simulink model "Accoppiato_percorso_lineare"  (R2020a)
settings: Solver=VariableStepAuto  StartTime=0.0  StopTime=1000  RelTol=1e-3
values from neighbouring files (symbols this model uses):
  Ag = 1    [completeLinearSimulation.m]
  Al = 1    [completeLinearSimulation.m]
  Cd = 1.2    [completeLinearSimulation.m]
  Cl = 0.3    [completeLinearSimulation.m]
  g = 9.81    [completeLinearSimulation.m]
  h = 1    [completeLinearSimulation.m]
  i_e = 100    [completeLinearSimulation.m]
  id1_ref = 0    [completeLinearSimulation.m]
  id2_ref = 0    [completeLinearSimulation.m]
  ig1_init = 0    [completeLinearSimulation.m]
  ig3_init = 0    [completeLinearSimulation.m]
  ig4_init = 0    [completeLinearSimulation.m]
  iq1_ref = (Fx1_ref)/((3/2)*(pi/tau)*(Ld*(M/Ld)*i_e))    (= 482.136730936)    [completeLinearSimulation.m]
  iq2_ref = (Fx2_ref)/((3/2)*(pi/tau)*(Ld*(M/Ld)*i_e))    (= 482.136730936)    [completeLinearSimulation.m]
  Jx = 296*10^3    (= 296000)    [completeLinearSimulation.m]
  Jy = 2853*10^3    (= 2853000)    [completeLinearSimulation.m]
  Jz = 2853*10^3    (= 2853000)    [completeLinearSimulation.m]
  Ky = lqr(Ay,By,Qy,Rry)    [completeLinearSimulation.m]
  Kz = lqr(Az,Bz,Qz,Rrz)    [completeLinearSimulation.m]
  l = 8    [completeLinearSimulation.m]
  Ld = 0.06    [completeLinearSimulation.m]
  Lq = 0.06    [completeLinearSimulation.m]
  M = 0.1    [completeLinearSimulation.m]
  m = 60000    [completeLinearSimulation.m]
  mu0 = 1.25*10^-6    (= 1.25e-06)    [completeLinearSimulation.m]
  Ng = 500    [completeLinearSimulation.m]
  Nr = 300    [completeLinearSimulation.m]
  p = 3    [completeLinearSimulation.m]
  PHI12 = eval(PHI)    [completeLinearSimulation.m]
  PHI20 = eval(PHI)    [completeLinearSimulation.m]
  PHI4 = eval(PHI)    [completeLinearSimulation.m]
  phi_init = 0    [completeLinearSimulation.m]
  PHIc = eval(int21)    [completeLinearSimulation.m]
  PHIf = eval(int11)    [completeLinearSimulation.m]
  PHIr = eval(int31)    [completeLinearSimulation.m]
  phiy = 0    [completeLinearSimulation.m]
  psi_init = 0    [completeLinearSimulation.m]
  ql_init = 0    [completeLinearSimulation.m]
  qv_init = 0    [completeLinearSimulation.m]
  Ra = 0    [completeLinearSimulation.m]
  radius = 0    [completeLinearSimulation.m]
  Rg = 100    [completeLinearSimulation.m]
  rho = 1.225    [completeLinearSimulation.m]
  Rx = 1.04    [completeLinearSimulation.m]
  Rz = 100    [completeLinearSimulation.m]
  Sa = 13    [completeLinearSimulation.m]
  Ss = 13    [completeLinearSimulation.m]
  tau = 1    [completeLinearSimulation.m]
  theta_init = 0    [completeLinearSimulation.m]
  vql_init = 0    [completeLinearSimulation.m]
  vqv_init = 0    [completeLinearSimulation.m]
  Vref_x = [Vq1_ref; Vd1_ref; Vq2_ref; Vd2_ref]    [completeLinearSimulation.m]
  Vref_y = [ Vg1; Vg2; Vg3; Vg4; Vg5; Vg6]    [completeLinearSimulation.m]
  Vref_z = [Vr1_ref; Vr2_ref; Vr3_ref; Vr4_ref; Vr5_ref; Vr6_ref]    [completeLinearSimulation.m]
  vx = 400/3.6    (= 111.111111111)    [completeLinearSimulation.m]
  vy_init = 0    [completeLinearSimulation.m]
  w = eval(omega_1)    [completeLinearSimulation.m]
  wpsi_init = 0    [completeLinearSimulation.m]
  xA = 12    [completeLinearSimulation.m]
  xB = 8    [completeLinearSimulation.m]
  Xref = [iq1_ref; id1_ref; iq2_ref; id2_ref; xdot_ref]    [completeLinearSimulation.m]
  y_init = 0.01    [completeLinearSimulation.m]
  yB = 2    [completeLinearSimulation.m]
  ymax = 0.02    [completeLinearSimulation.m]
  Yref = [y_ref; vy_ref; psi_ref; wpsi_ref; ig_ref; ig_ref; ig_ref; ig_ref; ig_ref; ig_ref; ql_ref; vql_ref]    [completeLinearSimulation.m]
  zA = 0.5    [completeLinearSimulation.m]
  zB = -0.5    [completeLinearSimulation.m]
  zi_rip = 0.05    [completeLinearSimulation.m]
  Zref = [z_ref zdot_ref phi_ref phidot_ref theta_ref thetadot_ref ir1_ref ir2_ref ir3_ref ir4_ref ir5_ref ir6_ref qv_ref vqv_ref].'    [completeLinearSimulation.m]
undefined symbols (not defined in the file or in its folder): Kx
settings Model: Creator=Federico  LastModifiedBy=Federico

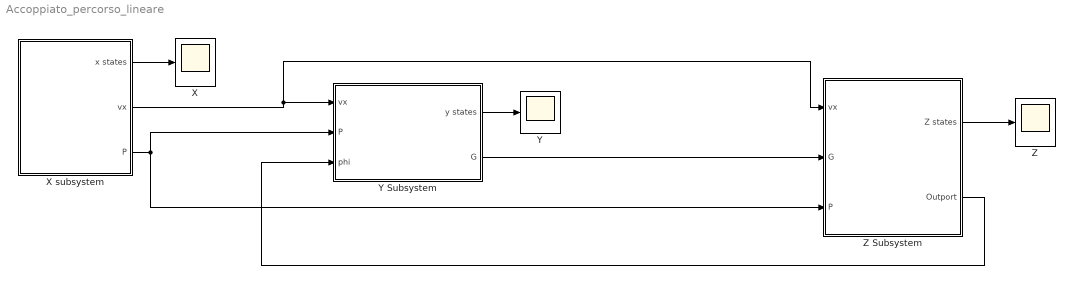
== system Accoppiato_percorso_lineare ==
  X : Scope
  X subsystem : Subsystem
  Y : Scope
  Y Subsystem : Subsystem
  Z : Scope
  Z Subsystem : Subsystem
  wires:
  X subsystem/1(x states) -> X/1
  X subsystem/3(P) -> Z Subsystem/3(P), Y Subsystem/2(P)
  X subsystem/2(vx) -> Z Subsystem/1(vx), Y Subsystem/1(vx)
  Y Subsystem/2(G) -> Z Subsystem/2(G)
  Y Subsystem/1(y states) -> Y/1
  Z Subsystem/1(Z states) -> Z/1
  Z Subsystem/2(Outport) -> Y Subsystem/3(phi)

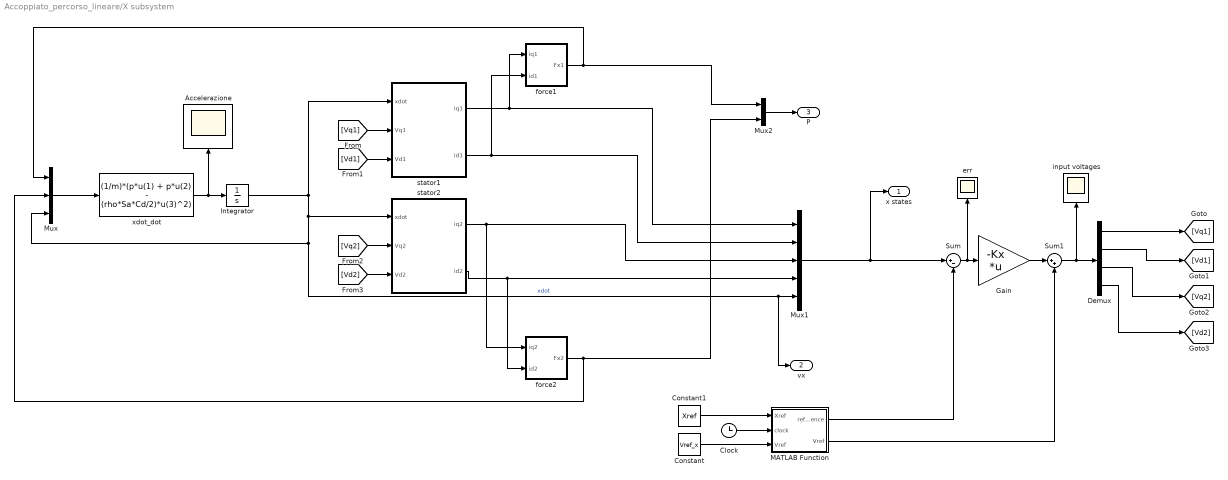
== system Accoppiato_percorso_lineare/X subsystem ==
  Accelerazione : Scope
  Clock : Clock
  Constant : Constant  Value=Vref_x
  Constant1 : Constant  Value=Xref
  Demux : Demux
  Gain : Gain  Gain=-Kx  Multiplication=Matrix(K*u)
  Integrator : Integrator
  MATLAB Function : MATLAB Function  TreatAsAtomicUnit=on
  Mux : Mux  Inputs=3
  Mux1 : Mux  Inputs=5
  Mux2 : Mux  Inputs=2
  Sum : Sum  Inputs=|+-
  Sum1 : Sum  Inputs=|++
  err : Scope
  force1 : Subsystem
  force2 : Subsystem
  input voltages : Scope
  stator1 : Subsystem
  stator2 : Subsystem
  xdot_dot : Fcn  Expr=(1/m)*(p*u(1) + p*u(2) - (rho*Sa*Cd/2)*u(3)^2)
  x states : Outport
  vx : Outport  Port=2
  P : Outport  Port=3
  wires:
  MATLAB Function/1(reference) -> Sum/2
  stator1/2(id1) -> Mux1/2, force1/2(id1)
  Sum1/1 -> Demux/1, input voltages/1
  Integrator/1 -> Mux/3, vx/1, Mux1/5, stator2/1(xdot), stator1/1(xdot)  "xdot"
  stator2/2(id2) -> force2/2(id2), Mux1/4
  [Vd2] -> stator2/3(Vd2)
  xdot_dot/1 -> Integrator/1, Accelerazione/1
  Demux/4 -> [Vd2]
  force1/1(Fx1) -> Mux2/1, Mux/1
  Mux1/1 -> Sum/1, x states/1
  Gain/1 -> Sum1/1
  MATLAB Function/2(Vref) -> Sum1/2
  Mux/1 -> xdot_dot/1
  Constant1/1 -> MATLAB Function/1(Xref)
  Sum/1 -> err/1, Gain/1
  Demux/1 -> [Vq1]
  stator1/1(iq1) -> Mux1/1, force1/1("iq1 ")
  Clock/1 -> MATLAB Function/2(clock)
  stator2/1(iq2) -> force2/1("iq2 "), Mux1/3
  Demux/3 -> [Vq2]
  [Vq2] -> stator2/2(Vq2)
  Constant/1 -> MATLAB Function/3("Vref ")
  Demux/2 -> [Vd1]
  [Vq1] -> stator1/2(Vq1)
  [Vd1] -> stator1/3(Vd1)
  force2/1(Fx2) -> Mux/2, Mux2/2
  Mux2/1 -> P/1

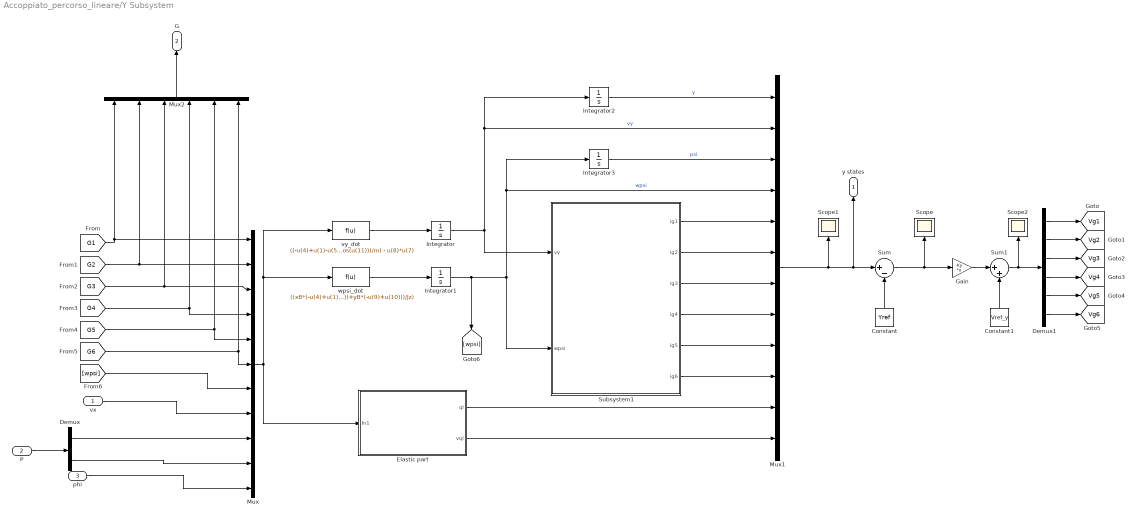
== system Accoppiato_percorso_lineare/Y Subsystem ==
  vx : Inport
  P : Inport  Port=2
  phi : Inport  Port=3
  Constant : Constant  Value=Yref
  Constant1 : Constant  Value=Vref_y
  Demux : Demux  Outputs=2
  Demux1 : Demux  Outputs=6
  Elastic part : Subsystem
  Gain : Gain  Gain=-Ky  Multiplication=Matrix(K*u)
  Integrator : Integrator  InitialCondition=vy_init
  Integrator1 : Integrator  InitialCondition=wpsi_init
  Integrator2 : Integrator  InitialCondition=y_init
  Integrator3 : Integrator  InitialCondition=psi_init
  Mux : Mux  Inputs=11
  Mux1 : Mux  Inputs=12
  Mux2 : Mux  Inputs=6
  Scope : Scope
  Scope1 : Scope
  Scope2 : Scope
  Subsystem1 : Subsystem
  Sum : Sum  Inputs=|+-
  Sum1 : Sum  Inputs=|++
  vy_dot : Fcn  Expr=((-u(4)+u(1)-u(5)+u(2)-u(6)+u(3)+m*g*sin(u(11))-m*Ra*(u(7)^2)*cos(u(11)))/m) - u(8)*u(7)
  wpsi_dot : Fcn  Expr=((xB*(-u(4)+u(1)+u(6)-u(3))+yB*(-u(9)+u(10)))/Jz)
  y states : Outport
  G : Outport  Port=2
  tag scope: Vg1=global, Vg2=global, Vg3=global, Vg4=global, Vg5=global, Vg6=global
  wires:
  Demux1/5 -> [Vg5]
  Integrator1/1 -> [wpsi], Integrator3/1, Mux1/4, Subsystem1/2(wpsi)  "wpsi"
  Demux1/4 -> [Vg4]
  [G2] -> Mux2/2, Mux/2
  Subsystem1/2(ig2) -> Mux1/6
  Mux/1 -> wpsi_dot/1, vy_dot/1, Elastic part/1(In1)
  Integrator3/1 -> Mux1/3  "psi"
  Gain/1 -> Sum1/1
  Subsystem1/1(ig1) -> Mux1/5
  Integrator/1 -> Integrator2/1, Mux1/2, Subsystem1/1(vy)  "vy"
  [G1] -> Mux2/1, Mux/1
  [G4] -> Mux2/4, Mux/4
  Constant/1 -> Sum/2
  Demux1/3 -> [Vg3]
  Subsystem1/4(ig4) -> Mux1/8
  Integrator2/1 -> Mux1/1  "y"
  Sum/1 -> Gain/1, Scope/1
  Demux1/1 -> [Vg1]
  Demux1/6 -> [Vg6]
  Subsystem1/5(ig5) -> Mux1/9
  Subsystem1/3(ig3) -> Mux1/7
  [G3] -> Mux2/3, Mux/3
  wpsi_dot/1 -> Integrator1/1
  Mux1/1 -> Sum/1, y states/1, Scope1/1
  Elastic part/1(ql) -> Mux1/11
  Constant1/1 -> Sum1/2
  Elastic part/2(vql) -> Mux1/12
  Sum1/1 -> Scope2/1, Demux1/1
  [G5] -> Mux2/5, Mux/5
  vy_dot/1 -> Integrator/1
  [G6] -> Mux2/6, Mux/6
  Demux1/2 -> [Vg2]
  Subsystem1/6(ig6) -> Mux1/10
  Mux2/1 -> G/1
  [wpsi] -> Mux/7
  vx/1 -> Mux/8
  Demux/1 -> Mux/9
  Demux/2 -> Mux/10
  P/1 -> Demux/1
  phi/1 -> Mux/11

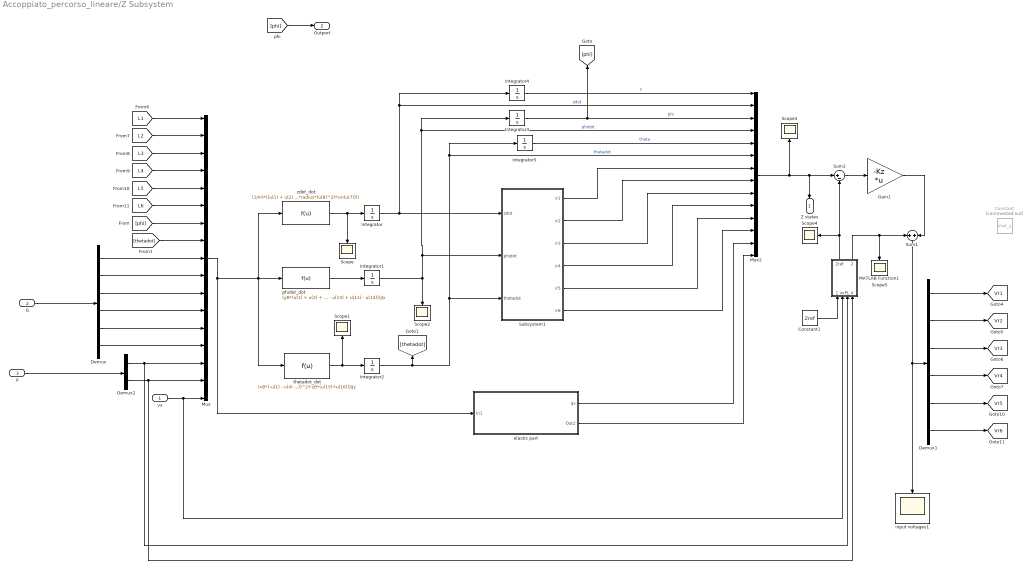
== system Accoppiato_percorso_lineare/Z Subsystem ==
  vx : Inport
  G : Inport  Port=2
  P : Inport  Port=3
  Constant : Constant  Commented=on  Value=Vref_z
  Constant1 : Constant  Value=Zref
  Demux : Demux  Outputs=6
  Demux1 : Demux  Outputs=6
  Demux2 : Demux  Outputs=2
  Gain1 : Gain  Gain=-Kz  Multiplication=Matrix(K*u)
  Integrator : Integrator
  Integrator1 : Integrator
  Integrator2 : Integrator
  Integrator3 : Integrator  InitialCondition=phi_init
  Integrator4 : Integrator  InitialCondition=h
  Integrator5 : Integrator  InitialCondition=theta_init
  MATLAB Function1 : MATLAB Function  TreatAsAtomicUnit=on
  Mux : Mux  Inputs=17
  Mux2 : Mux  Inputs=14
  Scope{,1..5} (6 alike) : Scope
  Subsystem1 : Subsystem
  Sum1 : Sum
  Sum2 : Sum  Inputs=|+-
  elastic part : Subsystem
  input voltages1 : Scope
  phidot_dot : Fcn  Expr=(yB*(u(1) + u(2) + u(3) - u(4) - u(5) - u(6)) + zB*(u(9) - u(12) + u(10) - u(13) + u(11) - u(14)))/Jx
  thetadot_dot : Fcn  Expr=(xB*(-u(1) - u(4) + u(3) + u(6)) -zA*(rho*Ss*Cd/2)*(u(17))^2+xA*(rho*Ss*Cl/2)*(u(17))^2+zB*(u(15)+u(16)))/Jy
  zdot_dot : Fcn  Expr=(1/m)*((u(1) + u(2) + u(3) + u(4) + u(5) + u(6) - (rho*Ss*Cl/2)*(u(17))^2 - m*g*cos(u(7)) - m*radius*(u(8)^2)*sin(u(7))))
  Z states : Outport
  Outport : Outport  Port=2
  tag scope: Vr1=global, Vr2=global, Vr3=global, Vr4=global, Vr5=global, Vr6=global
  wires:
  Sum1/1 -> Demux1/1, input voltages1/1
  elastic part/2(Out2) -> Mux2/14
  Mux/1 -> elastic part/1(In1), zdot_dot/1, phidot_dot/1, thetadot_dot/1
  [L3] -> Mux/3
  zdot_dot/1 -> Scope/1, Integrator/1
  [L5] -> Mux/5
  Integrator4/1 -> Mux2/1  "z"
  phidot_dot/1 -> Integrator1/1
  Mux2/1 -> Scope3/1, Z states/1, Sum2/1
  Sum2/1 -> Gain1/1
  Subsystem1/5(ir5) -> Mux2/11
  Subsystem1/2(ir2) -> Mux2/8
  Demux1/5 -> [Vr5]
  Demux1/1 -> [Vr1]
  Integrator2/1 -> Mux2/6, Integrator5/1, Subsystem1/3(thetadot), [thetadot]  "thetadot"
  [L6] -> Mux/6
  Integrator1/1 -> Scope2/1, Mux2/4, Integrator3/1, Subsystem1/2(phidot)  "phidot"
  [L2] -> Mux/2
  Demux1/4 -> [Vr4]
  elastic part/1(qv) -> Mux2/13
  Integrator3/1 -> [phi], Mux2/3  "phi"
  thetadot_dot/1 -> Integrator2/1, Scope1/1
  Subsystem1/6(ir6) -> Mux2/12
  Integrator5/1 -> Mux2/5  "theta"
  Integrator/1 -> Integrator4/1, Mux2/2, Subsystem1/1(zdot)  "zdot"
  [L4] -> Mux/4
  Subsystem1/3(ir3) -> Mux2/9
  Subsystem1/1(ir1) -> Mux2/7
  Demux1/2 -> [Vr2]
  Demux1/6 -> [Vr6]
  [L1] -> Mux/1
  Subsystem1/4(ir4) -> Mux2/10
  Demux1/3 -> [Vr3]
  [phi] -> Mux/7
  [thetadot] -> Mux/8
  G/1 -> Demux/1
  Demux/1 -> Mux/9
  Demux/2 -> Mux/10
  Demux/4 -> Mux/12
  Demux/3 -> Mux/11
  Demux/5 -> Mux/13
  Demux/6 -> Mux/14
  P/1 -> Demux2/1
  Demux2/1 -> MATLAB Function1/3(PL), Mux/15
  Demux2/2 -> MATLAB Function1/4(PR), Mux/16
  vx/1 -> MATLAB Function1/2(vx), Mux/17
  [phi] -> Outport/1
  Constant1/1 -> MATLAB Function1/1("Zref ")
  MATLAB Function1/1(Zref) -> Sum2/2, Scope4/1
  Gain1/1 -> Sum1/2
  MATLAB Function1/2(Vref_z) -> Sum1/1, Scope5/1

== system Accoppiato_percorso_lineare/X subsystem/force1 ==
  "iq1 " : Inport
  id1 : Inport  Port=2
  Fcn : Fcn  Expr=(3/2)*(pi/tau)*(Ld*((M/Ld)*i_e) + (Ld-Lq)*u(2))*u(1)
  Mux : Mux  Inputs=2
  Fx1 : Outport
  wires:
  Fcn/1 -> Fx1/1
  "iq1 "/1 -> Mux/1
  id1/1 -> Mux/2
  Mux/1 -> Fcn/1

== system Accoppiato_percorso_lineare/X subsystem/force2 ==
  "iq2 " : Inport
  id2 : Inport  Port=2
  Fcn : Fcn  Expr=(3/2)*(pi/tau)*(Ld*((M/Ld)*i_e) + (Ld-Lq)*u(2))*u(1)
  Mux : Mux  Inputs=2
  Fx2 : Outport
  wires:
  Fcn/1 -> Fx2/1
  "iq2 "/1 -> Mux/1
  id2/1 -> Mux/2
  Mux/1 -> Fcn/1

== system Accoppiato_percorso_lineare/X subsystem/stator1 ==
  xdot : Inport
  Vq1 : Inport  Port=2
  Vd1 : Inport  Port=3
  Integrator1 : Integrator  InitialCondition=iq1_ref
  Integrator2 : Integrator  InitialCondition=id1_ref
  Mux2 : Mux
  Mux3 : Mux
  id1_dot : Fcn  Expr=-(Rx/Ld)*u(4) - (Lq/Ld)*(u(3))*u(1)*pi/tau + u(2)/Ld
  iq1_dot : Fcn  Expr=-(Rx/Lq)*u(3) + (Ld/Lq)*((M/Ld)*i_e + u(4))*u(1)*pi/tau + u(2)/Lq
  iq1 : Outport
  id1 : Outport  Port=2
  wires:
  iq1_dot/1 -> Integrator1/1
  Mux3/1 -> id1_dot/1
  Mux2/1 -> iq1_dot/1
  Vd1/1 -> Mux3/2
  id1_dot/1 -> Integrator2/1
  xdot/1 -> Mux2/1, Mux3/1
  Integrator1/1 -> Mux2/3, Mux3/3, iq1/1  "iq1"
  Integrator2/1 -> Mux3/4, Mux2/4, id1/1  "id1"
  Vq1/1 -> Mux2/2

== system Accoppiato_percorso_lineare/X subsystem/stator2 ==
  xdot : Inport
  Vq2 : Inport  Port=2
  Vd2 : Inport  Port=3
  Integrator1 : Integrator  InitialCondition=iq2_ref
  Integrator2 : Integrator  InitialCondition=id2_ref
  Mux2 : Mux
  Mux3 : Mux
  id2_dot : Fcn  Expr=-(Rx/Ld)*u(4) - (Lq/Ld)*(u(3))*u(1)*pi/tau + u(2)/Ld
  iq2_dot : Fcn  Expr=-(Rx/Lq)*u(3) + (Ld/Lq)*((M/Ld)*i_e + u(4))*u(1)*pi/tau + u(2)/Lq
  iq2 : Outport
  id2 : Outport  Port=2
  wires:
  iq2_dot/1 -> Integrator1/1
  Mux3/1 -> id2_dot/1
  Mux2/1 -> iq2_dot/1
  Vd2/1 -> Mux3/2
  id2_dot/1 -> Integrator2/1
  xdot/1 -> Mux2/1, Mux3/1
  Integrator1/1 -> Mux2/3, Mux3/3, iq2/1  "iq2"
  Integrator2/1 -> Mux3/4, Mux2/4, id2/1  "id2"
  Vq2/1 -> Mux2/2

== system Accoppiato_percorso_lineare/Y Subsystem/Elastic part ==
  In1 : Inport
  From : From  Commented=on  GotoTag=ql  TagVisibility=global
  Integrator4 : Integrator  InitialCondition=vql_init
  Integrator5 : Integrator  InitialCondition=ql_init
  Mux2 : Mux
  gc : Fcn  Expr=(u(5)-u(2) +(m*g*sin(phiy)-m*radius*cos(phiy)*u(7)^2)/3)/l
  gf : Fcn  Expr=(u(4)-u(1) + (m*g*sin(phiy)-m*radius*cos(phiy)*u(7)^2)/3)/l
  gr : Fcn  Expr=(u(6)-u(3) +(m*g*sin(phiy)-m*radius*cos(phiy)*u(7)^2)/3)/l
  vql_dot : Fcn  Expr=-u(1)*(w^2) +(u(2)*PHIf)+(u(3)*PHIc)+(u(4)*PHIr)
  ql : Outport
  vql : Outport  Port=2
  tag scope: ql=global, vql=global
  wires:
  Integrator5/1 -> Mux2/1, [ql], ql/1  "ql"
  Integrator4/1 -> Integrator5/1, vql/1, [vql]  "vql"
  gr/1 -> Mux2/4
  In1/1 -> gr/1, gc/1, gf/1
  Mux2/1 -> vql_dot/1
  gf/1 -> Mux2/2
  gc/1 -> Mux2/3
  vql_dot/1 -> Integrator4/1

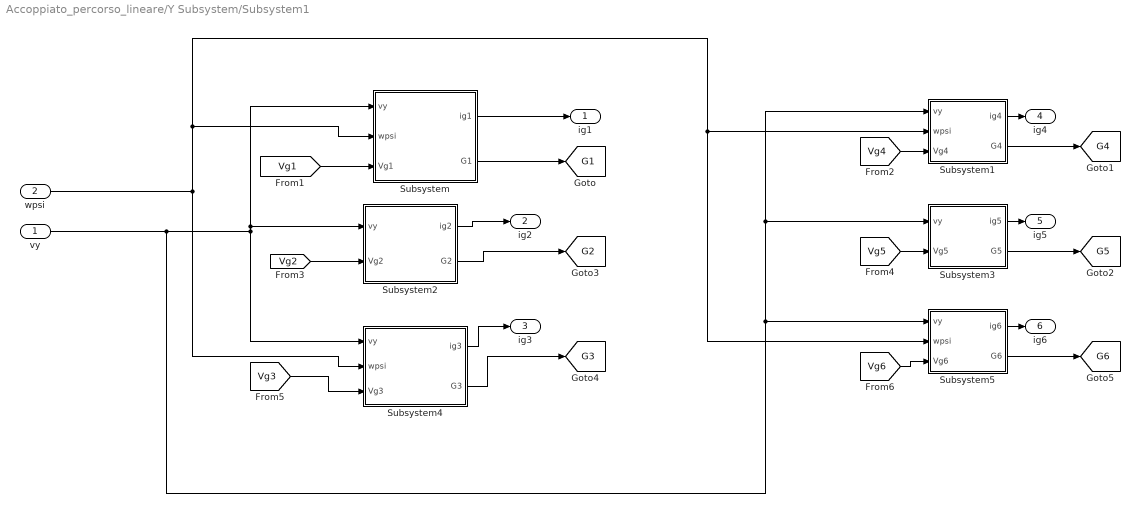
== system Accoppiato_percorso_lineare/Y Subsystem/Subsystem1 ==
  vy : Inport
  wpsi : Inport  Port=2
  Subsystem : Subsystem
  Subsystem1 : Subsystem
  Subsystem2 : Subsystem
  Subsystem3 : Subsystem
  Subsystem4 : Subsystem
  Subsystem5 : Subsystem
  ig1 : Outport
  ig2 : Outport  Port=2
  ig3 : Outport  Port=3
  ig4 : Outport  Port=4
  ig5 : Outport  Port=5
  ig6 : Outport  Port=6
  tag scope: G1=global, G2=global, G3=global, G4=global, G5=global, G6=global
  wires:
  Subsystem/2(G1) -> [G1]
  [Vg3] -> Subsystem4/3(Vg3)
  [Vg1] -> Subsystem/3(Vg1)
  Subsystem4/1(ig3) -> ig3/1
  Subsystem/1(ig1) -> ig1/1
  Subsystem2/1(ig2) -> ig2/1
  Subsystem2/2(G2) -> [G2]
  [Vg2] -> Subsystem2/2(Vg2)
  Subsystem4/2(G3) -> [G3]
  Subsystem5/2(G6) -> [G6]
  [Vg5] -> Subsystem3/2(Vg5)
  wpsi/1 -> Subsystem5/2(wpsi), Subsystem1/2(wpsi), Subsystem/2(wpsi), Subsystem4/2(wpsi)
  Subsystem3/2(G5) -> [G5]
  Subsystem3/1(ig5) -> ig5/1
  Subsystem1/1(ig4) -> ig4/1
  Subsystem5/1(ig6) -> ig6/1
  [Vg4] -> Subsystem1/3(Vg4)
  [Vg6] -> Subsystem5/3(Vg6)
  Subsystem1/2(G4) -> [G4]
  vy/1 -> Subsystem/1(vy), Subsystem2/1(vy), Subsystem4/1(vy), Subsystem1/1(vy), Subsystem3/1(vy), Subsystem5/1(vy)

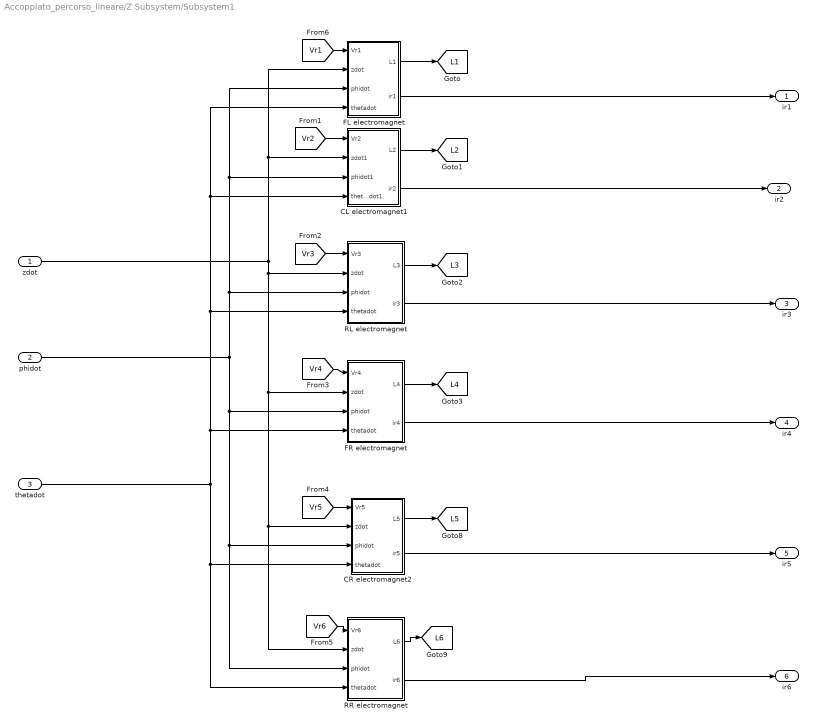
== system Accoppiato_percorso_lineare/Z Subsystem/Subsystem1 ==
  zdot : Inport
  phidot : Inport  Port=2
  thetadot : Inport  Port=3
  CL electromagnet1 : Subsystem
  CR electromagnet2 : Subsystem
  FL electromagnet : Subsystem
  FR electromagnet : Subsystem
  RL electromagnet : Subsystem
  RR electromagnet : Subsystem
  ir1 : Outport
  ir2 : Outport  Port=2
  ir3 : Outport  Port=3
  ir4 : Outport  Port=4
  ir5 : Outport  Port=5
  ir6 : Outport  Port=6
  tag scope: L1=global, L2=global, L3=global, L4=global, L5=global, L6=global
  wires:
  CL electromagnet1/2(ir2) -> ir2/1
  [Vr3] -> RL electromagnet/1(Vr3)
  FR electromagnet/1(L4) -> [L4]
  CL electromagnet1/1(L2) -> [L2]
  FL electromagnet/1(L1) -> [L1]
  RR electromagnet/1(L6) -> [L6]
  CR electromagnet2/1(L5) -> [L5]
  [Vr6] -> RR electromagnet/1(Vr6)
  phidot/1 -> FR electromagnet/3(phidot), RR electromagnet/3(phidot), CR electromagnet2/3(phidot), FL electromagnet/3(phidot), CL electromagnet1/3(phidot1), RL electromagnet/3(phidot)
  [Vr4] -> FR electromagnet/1(Vr4)
  FR electromagnet/2(ir4) -> ir4/1
  zdot/1 -> CL electromagnet1/2(zdot1), FL electromagnet/2(zdot), RL electromagnet/2(zdot), FR electromagnet/2(zdot), RR electromagnet/2(zdot), CR electromagnet2/2(zdot)
  RL electromagnet/2(ir3) -> ir3/1
  FL electromagnet/2(ir1) -> ir1/1
  [Vr2] -> CL electromagnet1/1(Vr2)
  thetadot/1 -> RR electromagnet/4(thetadot), CR electromagnet2/4(thetadot), FL electromagnet/4(thetadot), CL electromagnet1/4(thetadot1), RL electromagnet/4(thetadot), FR electromagnet/4(thetadot)
  CR electromagnet2/2(ir5) -> ir5/1
  [Vr5] -> CR electromagnet2/1(Vr5)
  RR electromagnet/2(ir6) -> ir6/1
  RL electromagnet/1(L3) -> [L3]
  [Vr1] -> FL electromagnet/1(Vr1)

== system Accoppiato_percorso_lineare/Z Subsystem/elastic part ==
  In1 : Inport
  Integrator6 : Integrator  InitialCondition=vqv_init
  Integrator7 : Integrator  InitialCondition=qv_init
  Mux1 : Mux
  lc : Fcn  Expr=(u(3)+u(4)-((rho*Ss*Cl/2)*(vx)^2+m*radius*(u(8)^2)*sin(u(7))+m*g*cos(u(7)))/3)/l
  lf : Fcn  Expr=(u(1)+u(2)-((rho*Ss*Cl/2)*(vx)^2+m*radius*(u(8)^2)*sin(u(7))+m*g*cos(u(7)))/3)/l
  lr : Fcn  Expr=(u(5)+u(6)-((rho*Ss*Cl/2)*(vx)^2+m*radius*(u(8)^2)*sin(u(7))+m*g*cos(u(7)))/3)/l
  vqv_dot : Fcn  Expr=-u(1)*w^2+u(2)*PHIf+u(3)*PHIc+u(4)*PHIr
  qv : Outport
  Out2 : Outport  Port=2
  tag scope: qv=global, vqv=global
  wires:
  In1/1 -> lc/1, lr/1, lf/1
  Mux1/1 -> vqv_dot/1
  lf/1 -> Mux1/2
  vqv_dot/1 -> Integrator6/1
  Integrator7/1 -> qv/1, [qv], Mux1/1  "qv"
  lc/1 -> Mux1/3
  Integrator6/1 -> Out2/1, [vqv], Integrator7/1  "vqv"
  lr/1 -> Mux1/4

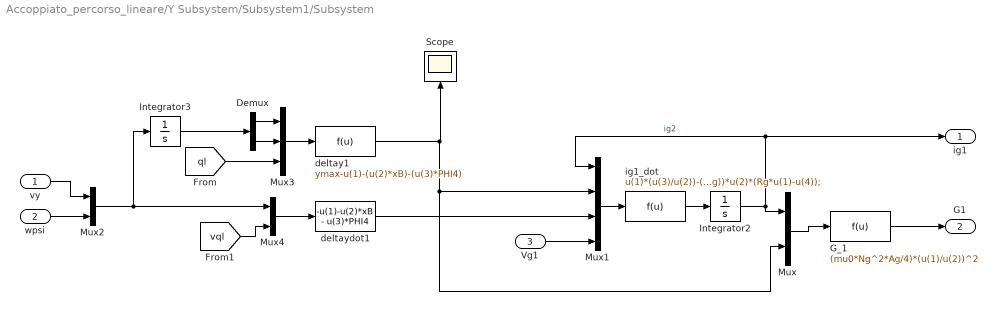
== system Accoppiato_percorso_lineare/Y Subsystem/Subsystem1/Subsystem ==
  vy : Inport
  wpsi : Inport  Port=2
  Vg1 : Inport  Port=3
  Demux : Demux  Outputs=2
  G_1 : Fcn  Expr=(mu0*Ng^2*Ag/4)*(u(1)/u(2))^2
  Integrator2 : Integrator  InitialCondition=ig1_init
  Integrator3 : Integrator  InitialCondition=[y_init; psi_init]
  Mux : Mux  Inputs=2
  Mux1 : Mux
  Mux2 : Mux  Inputs=2
  Mux3 : Mux  Inputs=3
  Mux4 : Mux  Inputs=2
  Scope : Scope
  deltay1 : Fcn  Expr=ymax-u(1)-(u(2)*xB)-(u(3)*PHI4)
  deltaydot1 : Fcn  Expr=-u(1)-u(2)*xB - u(3)*PHI4
  ig1_dot : Fcn  Expr=u(1)*(u(3)/u(2))-(2/(mu0*(Ng^2)*Ag))*u(2)*(Rg*u(1)-u(4));
  ig1 : Outport
  G1 : Outport  Port=2
  wires:
  ig1_dot/1 -> Integrator2/1
  G_1/1 -> G1/1
  deltaydot1/1 -> Mux1/3
  vy/1 -> Mux2/1
  Mux2/1 -> Mux4/1, Integrator3/1
  Vg1/1 -> Mux1/4
  Mux/1 -> G_1/1
  Integrator2/1 -> Mux/1, ig1/1, Mux1/1  "ig2"
  wpsi/1 -> Mux2/2
  Mux1/1 -> ig1_dot/1
  deltay1/1 -> Mux1/2, Mux/2, Scope/1
  Mux3/1 -> deltay1/1
  Mux4/1 -> deltaydot1/1
  [ql] -> Mux3/3
  [vql] -> Mux4/2
  Integrator3/1 -> Demux/1
  Demux/1 -> Mux3/1
  Demux/2 -> Mux3/2

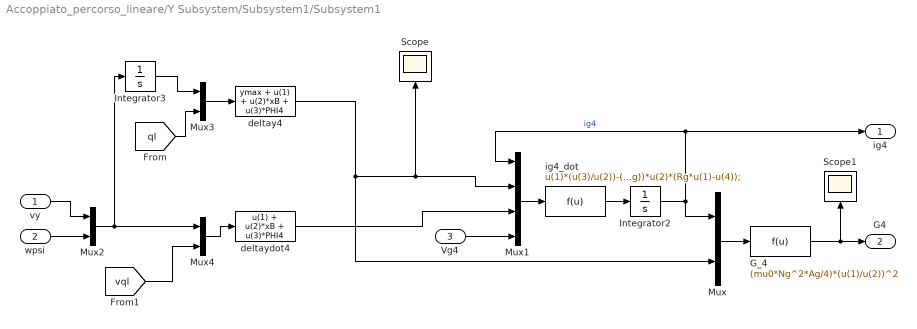
== system Accoppiato_percorso_lineare/Y Subsystem/Subsystem1/Subsystem1 ==
  vy : Inport
  wpsi : Inport  Port=2
  Vg4 : Inport  Port=3
  G_4 : Fcn  Expr=(mu0*Ng^2*Ag/4)*(u(1)/u(2))^2
  Integrator2 : Integrator  InitialCondition=ig1_init
  Integrator3 : Integrator  InitialCondition=[y_init; psi_init]
  Mux{,2..4} (4 alike) : Mux  Inputs=2
  Mux1 : Mux
  Scope : Scope
  Scope1 : Scope
  deltay4 : Fcn  Expr=ymax + u(1) + u(2)*xB + u(3)*PHI4
  deltaydot4 : Fcn  Expr=u(1) + u(2)*xB + u(3)*PHI4
  ig4_dot : Fcn  Expr=u(1)*(u(3)/u(2))-(2/(mu0*(Ng^2)*Ag))*u(2)*(Rg*u(1)-u(4));
  ig4 : Outport
  G4 : Outport  Port=2
  wires:
  deltay4/1 -> Mux/2, Mux1/2, Scope/1
  Mux1/1 -> ig4_dot/1
  wpsi/1 -> Mux2/2
  Integrator2/1 -> Mux1/1, ig4/1, Mux/1  "ig4"
  Mux/1 -> G_4/1
  Vg4/1 -> Mux1/4
  Mux2/1 -> Mux4/1, Integrator3/1
  vy/1 -> Mux2/1
  deltaydot4/1 -> Mux1/3
  G_4/1 -> Scope1/1, G4/1
  ig4_dot/1 -> Integrator2/1
  Integrator3/1 -> Mux3/1
  Mux3/1 -> deltay4/1
  [ql] -> Mux3/2
  Mux4/1 -> deltaydot4/1
  [vql] -> Mux4/2

== system Accoppiato_percorso_lineare/Y Subsystem/Subsystem1/Subsystem2 ==
  vy : Inport
  Vg2 : Inport  Port=2
  G_2 : Fcn  Expr=(mu0*Ng^2*Ag/4)*(u(1)/u(2))^2
  Integrator2 : Integrator  InitialCondition=ig4_init
  Integrator3 : Integrator  InitialCondition=y_init
  Mux : Mux  Inputs=2
  Mux1 : Mux
  Mux2 : Mux  Inputs=2
  Mux3 : Mux  Inputs=2
  deltay2 : Fcn  Expr=ymax - u(1) - u(2)*PHI12
  deltaydot2 : Fcn  Expr=-u(1) - u(2)*PHI12
  ig2_dot : Fcn  Expr=u(1)*u(3)/u(2)-(2/(mu0*(Ng^2)*Ag))*u(2)*(Rg*u(1)-u(4));
  ig2 : Outport
  G2 : Outport  Port=2
  wires:
  deltay2/1 -> Mux/2, Mux1/2
  Mux1/1 -> ig2_dot/1
  Integrator2/1 -> Mux/1, Mux1/1, ig2/1  "ig2"
  Mux/1 -> G_2/1
  Vg2/1 -> Mux1/4
  deltaydot2/1 -> Mux1/3
  G_2/1 -> G2/1
  ig2_dot/1 -> Integrator2/1
  vy/1 -> Mux3/1, Integrator3/1
  Mux2/1 -> deltay2/1
  Integrator3/1 -> Mux2/1
  [ql] -> Mux2/2
  Mux3/1 -> deltaydot2/1
  [vql] -> Mux3/2

== system Accoppiato_percorso_lineare/Y Subsystem/Subsystem1/Subsystem3 ==
  vy : Inport
  Vg5 : Inport  Port=2
  G_5 : Fcn  Expr=(mu0*Ng^2*Ag/4)*(u(1)/u(2))^2
  Integrator2 : Integrator  InitialCondition=ig4_init
  Integrator3 : Integrator  InitialCondition=y_init
  Mux : Mux  Inputs=2
  Mux1 : Mux
  Mux2 : Mux  Inputs=2
  Mux3 : Mux  Inputs=2
  deltay5 : Fcn  Expr=ymax + u(1) + u(2)*PHI12
  deltaydot5 : Fcn  Expr=u(1)+u(2)*PHI12
  ig5_dot : Fcn  Expr=u(1)*u(3)/u(2)-(2/(mu0*(Ng^2)*Ag))*u(2)*(Rg*u(1)-u(4));
  ig5 : Outport
  G5 : Outport  Port=2
  wires:
  vy/1 -> Mux3/1, Integrator3/1
  ig5_dot/1 -> Integrator2/1
  G_5/1 -> G5/1
  deltaydot5/1 -> Mux1/3
  Vg5/1 -> Mux1/4
  Mux/1 -> G_5/1
  Integrator2/1 -> ig5/1, Mux1/1, Mux/1  "ig5"
  Mux1/1 -> ig5_dot/1
  deltay5/1 -> Mux/2, Mux1/2
  Integrator3/1 -> Mux2/1
  Mux2/1 -> deltay5/1
  [ql] -> Mux2/2
  Mux3/1 -> deltaydot5/1
  [vql] -> Mux3/2

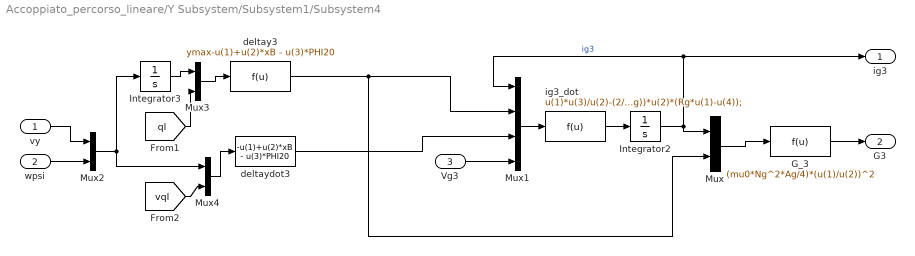
== system Accoppiato_percorso_lineare/Y Subsystem/Subsystem1/Subsystem4 ==
  vy : Inport
  wpsi : Inport  Port=2
  Vg3 : Inport  Port=3
  G_3 : Fcn  Expr=(mu0*Ng^2*Ag/4)*(u(1)/u(2))^2
  Integrator2 : Integrator  InitialCondition=ig3_init
  Integrator3 : Integrator  InitialCondition=[y_init; psi_init]
  Mux{,2..4} (4 alike) : Mux  Inputs=2
  Mux1 : Mux
  deltay3 : Fcn  Expr=ymax-u(1)+u(2)*xB - u(3)*PHI20
  deltaydot3 : Fcn  Expr=-u(1)+u(2)*xB - u(3)*PHI20
  ig3_dot : Fcn  Expr=u(1)*u(3)/u(2)-(2/(mu0*(Ng^2)*Ag))*u(2)*(Rg*u(1)-u(4));
  ig3 : Outport
  G3 : Outport  Port=2
  wires:
  ig3_dot/1 -> Integrator2/1
  G_3/1 -> G3/1
  deltaydot3/1 -> Mux1/3
  vy/1 -> Mux2/1
  Mux2/1 -> Integrator3/1, Mux4/1
  Vg3/1 -> Mux1/4
  Mux/1 -> G_3/1
  Integrator2/1 -> ig3/1, Mux1/1, Mux/1  "ig3"
  wpsi/1 -> Mux2/2
  deltay3/1 -> Mux/2, Mux1/2
  Mux1/1 -> ig3_dot/1
  Mux3/1 -> deltay3/1
  Integrator3/1 -> Mux3/1
  [ql] -> Mux3/2
  [vql] -> Mux4/2
  Mux4/1 -> deltaydot3/1

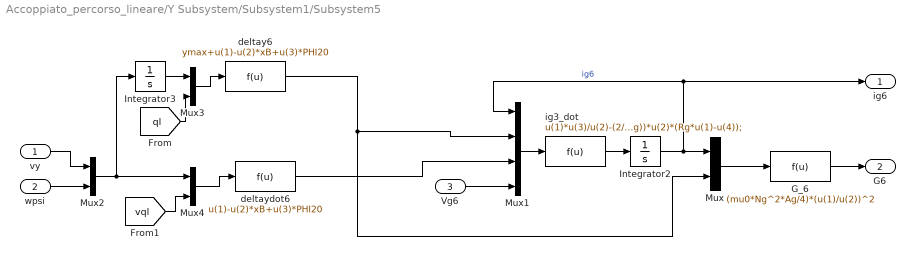
== system Accoppiato_percorso_lineare/Y Subsystem/Subsystem1/Subsystem5 ==
  vy : Inport
  wpsi : Inport  Port=2
  Vg6 : Inport  Port=3
  G_6 : Fcn  Expr=(mu0*Ng^2*Ag/4)*(u(1)/u(2))^2
  Integrator2 : Integrator  InitialCondition=ig3_init
  Integrator3 : Integrator  InitialCondition=[y_init; psi_init]
  Mux{,2..4} (4 alike) : Mux  Inputs=2
  Mux1 : Mux
  deltay6 : Fcn  Expr=ymax+u(1)-u(2)*xB+u(3)*PHI20
  deltaydot6 : Fcn  Expr=u(1)-u(2)*xB+u(3)*PHI20
  ig3_dot : Fcn  Expr=u(1)*u(3)/u(2)-(2/(mu0*(Ng^2)*Ag))*u(2)*(Rg*u(1)-u(4));
  ig6 : Outport
  G6 : Outport  Port=2
  wires:
  deltay6/1 -> Mux/2, Mux1/2
  Integrator3/1 -> Mux3/1
  Mux1/1 -> ig3_dot/1
  wpsi/1 -> Mux2/2
  Integrator2/1 -> Mux/1, Mux1/1, ig6/1  "ig6"
  Mux/1 -> G_6/1
  Vg6/1 -> Mux1/4
  Mux2/1 -> Integrator3/1, Mux4/1
  vy/1 -> Mux2/1
  deltaydot6/1 -> Mux1/3
  G_6/1 -> G6/1
  ig3_dot/1 -> Integrator2/1
  Mux3/1 -> deltay6/1
  [ql] -> Mux3/2
  Mux4/1 -> deltaydot6/1
  [vql] -> Mux4/2

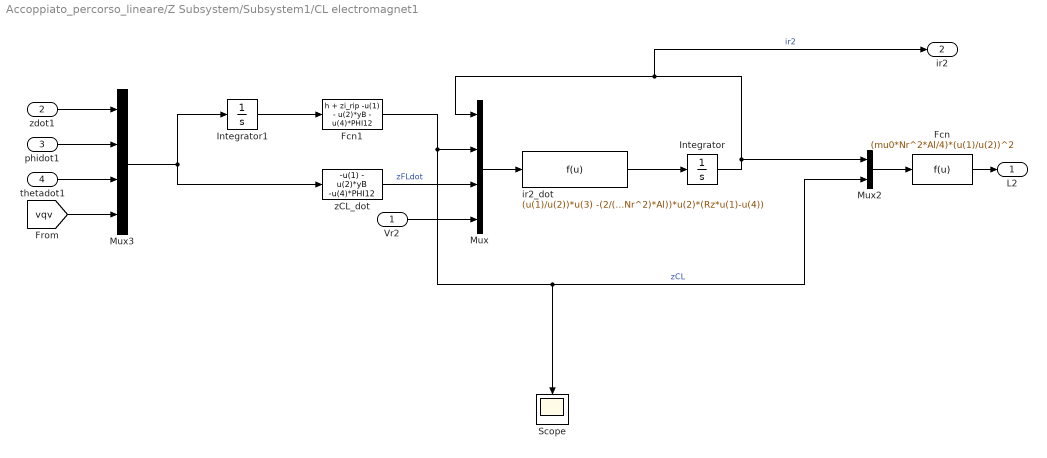
== system Accoppiato_percorso_lineare/Z Subsystem/Subsystem1/CL electromagnet1 ==
  Vr2 : Inport
  zdot1 : Inport  Port=2
  phidot1 : Inport  Port=3
  thetadot1 : Inport  Port=4
  Fcn : Fcn  Expr=(mu0*Nr^2*Al/4)*(u(1)/u(2))^2
  Fcn1 : Fcn  Expr=h + zi_rip -u(1) - u(2)*yB - u(4)*PHI12
  Integrator : Integrator
  Integrator1 : Integrator  InitialCondition=[h; phi_init; theta_init;qv_init]
  Mux : Mux
  Mux2 : Mux  Inputs=2
  Mux3 : Mux
  Scope : Scope
  ir2_dot : Fcn  Expr=(u(1)/u(2))*u(3) -(2/(mu0*(Nr^2)*Al))*u(2)*(Rz*u(1)-u(4))
  zCL_dot : Fcn  Expr=-u(1) - u(2)*yB -u(4)*PHI12
  L2 : Outport
  ir2 : Outport  Port=2
  wires:
  Mux/1 -> ir2_dot/1
  Vr2/1 -> Mux/4
  ir2_dot/1 -> Integrator/1
  Integrator/1 -> Mux2/1, ir2/1, Mux/1  "ir2"
  zCL_dot/1 -> Mux/3  "zFLdot"
  Fcn1/1 -> Scope/1, Mux2/2, Mux/2  "zCL"
  Mux2/1 -> Fcn/1
  Fcn/1 -> L2/1
  Integrator1/1 -> Fcn1/1
  thetadot1/1 -> Mux3/3
  phidot1/1 -> Mux3/2
  zdot1/1 -> Mux3/1
  [vqv] -> Mux3/4
  Mux3/1 -> zCL_dot/1, Integrator1/1

== system Accoppiato_percorso_lineare/Z Subsystem/Subsystem1/CR electromagnet2 ==
  Vr5 : Inport
  zdot : Inport  Port=2
  phidot : Inport  Port=3
  thetadot : Inport  Port=4
  Fcn : Fcn  Expr=(mu0*Nr^2*Al/4)*(u(1)/u(2))^2
  Fcn1 : Fcn  Expr=h + zi_rip - u(1) + u(2)*yB -u(4)*PHI12
  Integrator : Integrator
  Integrator1 : Integrator  InitialCondition=[h; phi_init; theta_init;qv_init]
  Mux : Mux
  Mux1 : Mux
  Mux2 : Mux  Inputs=2
  ir5_dot : Fcn  Expr=(u(1)/u(2))*u(3) -(2/(mu0*(Nr^2)*Al))*u(2)*(Rz*u(1)-u(4))
  zCR_dot : Fcn  Expr=-u(1) + u(2)*yB - u(4)*PHI12
  L5 : Outport
  ir5 : Outport  Port=2
  wires:
  Mux/1 -> ir5_dot/1
  Vr5/1 -> Mux/4
  ir5_dot/1 -> Integrator/1
  Integrator/1 -> Mux2/1, ir5/1, Mux/1  "ir5"
  zCR_dot/1 -> Mux/3  "zCRdot"
  Fcn1/1 -> Mux2/2, Mux/2  "zCR"
  Mux2/1 -> Fcn/1
  Fcn/1 -> L5/1
  Integrator1/1 -> Fcn1/1
  thetadot/1 -> Mux1/3
  phidot/1 -> Mux1/2
  zdot/1 -> Mux1/1
  [vqv] -> Mux1/4
  Mux1/1 -> Integrator1/1, zCR_dot/1

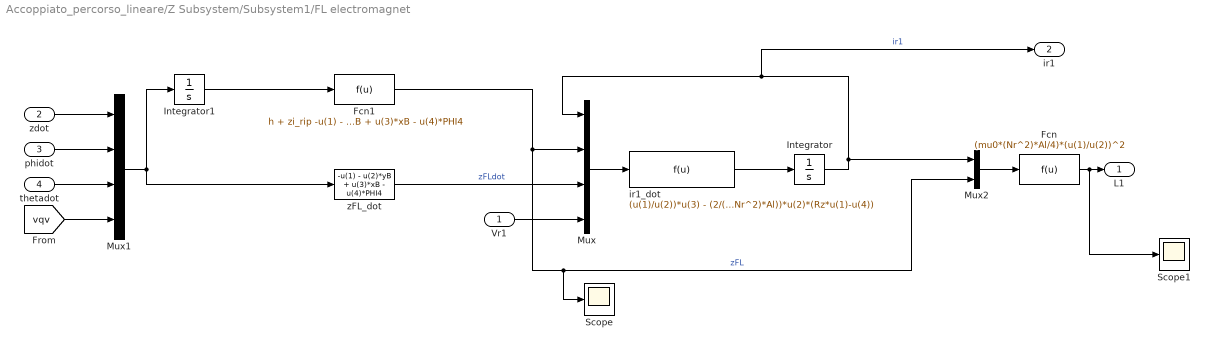
== system Accoppiato_percorso_lineare/Z Subsystem/Subsystem1/FL electromagnet ==
  Vr1 : Inport
  zdot : Inport  Port=2
  phidot : Inport  Port=3
  thetadot : Inport  Port=4
  Fcn : Fcn  Expr=(mu0*(Nr^2)*Al/4)*(u(1)/u(2))^2
  Fcn1 : Fcn  Expr=h + zi_rip -u(1) - u(2)*yB + u(3)*xB - u(4)*PHI4
  Integrator : Integrator
  Integrator1 : Integrator  InitialCondition=[h; phi_init; theta_init; qv_init]
  Mux : Mux
  Mux1 : Mux
  Mux2 : Mux  Inputs=2
  Scope : Scope
  Scope1 : Scope
  ir1_dot : Fcn  Expr=(u(1)/u(2))*u(3) - (2/(mu0*(Nr^2)*Al))*u(2)*(Rz*u(1)-u(4))
  zFL_dot : Fcn  Expr=-u(1) - u(2)*yB + u(3)*xB - u(4)*PHI4
  L1 : Outport
  ir1 : Outport  Port=2
  wires:
  Mux/1 -> ir1_dot/1
  Vr1/1 -> Mux/4
  ir1_dot/1 -> Integrator/1
  Integrator/1 -> Mux2/1, ir1/1, Mux/1  "ir1"
  Mux1/1 -> Integrator1/1, zFL_dot/1
  zdot/1 -> Mux1/1
  phidot/1 -> Mux1/2
  thetadot/1 -> Mux1/3
  zFL_dot/1 -> Mux/3  "zFLdot"
  Fcn1/1 -> Scope/1, Mux2/2, Mux/2  "zFL"
  Mux2/1 -> Fcn/1
  Fcn/1 -> Scope1/1, L1/1
  Integrator1/1 -> Fcn1/1
  [vqv] -> Mux1/4

== system Accoppiato_percorso_lineare/Z Subsystem/Subsystem1/FR electromagnet ==
  Vr4 : Inport
  zdot : Inport  Port=2
  phidot : Inport  Port=3
  thetadot : Inport  Port=4
  Fcn : Fcn  Expr=(mu0*Nr^2*Al/4)*(u(1)/u(2))^2
  Fcn1 : Fcn  Expr=h + zi_rip - u(1) + u(2)*yB + u(3)*xB - u(4)*PHI4
  Integrator : Integrator
  Integrator1 : Integrator  InitialCondition=[h; phi_init; theta_init;qv_init]
  Mux : Mux
  Mux1 : Mux
  Mux2 : Mux  Inputs=2
  ir4_dot : Fcn  Expr=(u(1)/u(2))*u(3) -(2/(mu0*(Nr^2)*Al))*u(2)*(Rz*u(1)-u(4))
  zFR_dot : Fcn  Expr=-u(1) + u(2)*yB + u(3)*xB - u(4)*PHI4
  L4 : Outport
  ir4 : Outport  Port=2
  wires:
  Mux/1 -> ir4_dot/1
  Vr4/1 -> Mux/4
  ir4_dot/1 -> Integrator/1
  zFR_dot/1 -> Mux/3  "zFLdot"
  Fcn1/1 -> Mux2/2, Mux/2  "zFR"
  Mux2/1 -> Fcn/1
  Fcn/1 -> L4/1
  Integrator/1 -> Mux2/1, ir4/1, Mux/1  "ir4"
  Integrator1/1 -> Fcn1/1
  thetadot/1 -> Mux1/3
  phidot/1 -> Mux1/2
  zdot/1 -> Mux1/1
  [vqv] -> Mux1/4
  Mux1/1 -> zFR_dot/1, Integrator1/1

== system Accoppiato_percorso_lineare/Z Subsystem/Subsystem1/RL electromagnet ==
  Vr3 : Inport
  zdot : Inport  Port=2
  phidot : Inport  Port=3
  thetadot : Inport  Port=4
  Fcn : Fcn  Expr=(mu0*Nr^2*Al/4)*(u(1)/u(2))^2
  Fcn1 : Fcn  Expr=h + zi_rip -u(1) - u(2)*yB - u(3)*xB - u(4)*PHI20
  Integrator : Integrator
  Integrator1 : Integrator  InitialCondition=[h; phi_init; theta_init;qv_init]
  Mux : Mux
  Mux1 : Mux
  Mux2 : Mux  Inputs=2
  Scope : Scope
  ir3_dot : Fcn  Expr=(u(1)/u(2))*u(3) -(2/(mu0*(Nr^2)*Al))*u(2)*(Rz*u(1)-u(4))
  zRL_dot : Fcn  Expr=-u(1) - u(2)*yB - u(3)*xB - u(4)*PHI20
  L3 : Outport
  ir3 : Outport  Port=2
  wires:
  Mux/1 -> ir3_dot/1
  Vr3/1 -> Mux/4
  ir3_dot/1 -> Integrator/1
  zRL_dot/1 -> Mux/3  "zFLdot"
  Fcn1/1 -> Scope/1, Mux2/2, Mux/2  "zRL"
  Mux2/1 -> Fcn/1
  Fcn/1 -> L3/1
  Integrator/1 -> Mux2/1, ir3/1, Mux/1  "ir1"
  Integrator1/1 -> Fcn1/1
  thetadot/1 -> Mux1/3
  phidot/1 -> Mux1/2
  zdot/1 -> Mux1/1
  [vqv] -> Mux1/4
  Mux1/1 -> zRL_dot/1, Integrator1/1

== system Accoppiato_percorso_lineare/Z Subsystem/Subsystem1/RR electromagnet ==
  Vr6 : Inport
  zdot : Inport  Port=2
  phidot : Inport  Port=3
  thetadot : Inport  Port=4
  Fcn : Fcn  Expr=(mu0*Nr^2*Al/4)*(u(1)/u(2))^2
  Fcn1 : Fcn  Expr=h + zi_rip - u(1) + u(2)*yB - u(3)*xB - u(4)*PHI20
  Integrator : Integrator
  Integrator1 : Integrator  InitialCondition=[h; phi_init; theta_init;qv_init]
  Mux : Mux
  Mux1 : Mux
  Mux2 : Mux  Inputs=2
  ir6_dot : Fcn  Expr=(u(1)/u(2))*u(3) -(2/(mu0*(Nr^2)*Al))*u(2)*(Rz*u(1)-u(4))
  zRR_dot : Fcn  Expr=-u(1) + u(2)*yB - u(3)*xB - u(4)*PHI20
  L6 : Outport
  ir6 : Outport  Port=2
  wires:
  Mux/1 -> ir6_dot/1
  Vr6/1 -> Mux/4
  ir6_dot/1 -> Integrator/1
  zRR_dot/1 -> Mux/3  "zFLdot"
  Fcn1/1 -> Mux2/2, Mux/2  "zRR"
  Mux2/1 -> Fcn/1
  Fcn/1 -> L6/1
  Integrator/1 -> Mux2/1, ir6/1, Mux/1  "ir6"
  Integrator1/1 -> Fcn1/1
  thetadot/1 -> Mux1/3
  phidot/1 -> Mux1/2
  zdot/1 -> Mux1/1
  [vqv] -> Mux1/4
  Mux1/1 -> Integrator1/1, zRR_dot/1

== matlab function Accoppiato_percorso_lineare/X subsystem/MATLAB Function ==
  data: Xref input; reference output; clock input; Vref output; Vref input
function [reference,Vref]= fcn(Xref,clock,Vref)
%% Solo Accelerazione
% steadyTime = 220; %più o meno come quello del paper mandato da luca. Comunque l'accelerazione sembra rimanere molto contenuta
% t = clock;
% 
% if t <= steadyTime
%     ramp = (1/steadyTime)*t;
% else
%     ramp = 1;
% end
% 
% % reference(5)=reference(5)*ramp; % Questo fa crescere sotto forma di rampa
% % solamente la velocità
% reference = Xref*ramp; %con questo tutte le grandezze crescono come una rampa nel tempo, tende a rendere leggermente più lento l'aumento della velocità ma non è troppo evidente
% Vref=Vref*ramp;
%% Accelerazione + decelerazione

%profilo trapezoidale per la velocità
%Ogni volta che si accelera decelera o altro viene introdotto un ritardo di
%x secondi. Questo ritardo dipende dal valore di i_e che nel nostro caso lavora come disturbo,
%se i_e=100 il ritardo è di circa 20 secondi quindi se voglio accelerare per 220 secondi setadyTime 
%dev'essere uguale a 200 e lo stesso vale per gli altri valori
steadyTime = 200; %più o meno come quello del paper mandato da luca. Comunque l'accelerazione sembra rimanere molto contenuta
crocera = 180; %secondi in cui il treno va a massima velocità
decelerazione = 180; % secondi necessari alla decelerazione del treno
t = clock; % tempo della simulazione

if t <= steadyTime
    ramp = (1/steadyTime)*t;
elseif and(t > steadyTime, t< steadyTime + crocera)
    ramp = 1;
elseif and(t >= steadyTime + crocera,t <= steadyTime + crocera + decelerazione)
    ramp = 1 - (1/decelerazione)*(t -(steadyTime + crocera));
else
    ramp = 0;
end

reference = Xref*ramp; %con questo tutte le grandezze crescono come una rampa nel tempo, tende a rendere leggermente più lento l'aumento della velocità ma non è troppo evidente

Vref=Vref*ramp;

== matlab function Accoppiato_percorso_lineare/Z Subsystem/MATLAB Function1 ==
  data: Zref input; Zref output; vx input; PL input; PR input; Vref_z output
function [Zref,Vref_z]= fcn(Zref,vx,PL,PR)

zi_ref = 0.01;
m = 60000;
xB=8;
zB=-0.5;
mu0=1.25*10^-6;
Nr=300;
Al=1;
rho=1.225;
Ss=13;
Cd=1.2;
Cl=0.3;
g=9.81;
Rz=100;
xA=12;
zA=0.5;

iri_ref = sqrt( (1/(6*(mu0*Nr^2*Al/4)))*((rho*Ss*Cl/2)*(vx)^2 + m*g)*zi_ref^2);
L2_ref = (mu0*Nr^2*Al/4)*(iri_ref/zi_ref)^2;
L5_ref = L2_ref;
L1_ref = -(1/2)*L2_ref -(1/4)*((zA/xB)*(rho*Ss*Cd/2)*vx^2 - (xA/xB)*(rho*Ss*Cl/2)*vx^2 - (zB/xB)*(PL+PR)) + (1/4)*(rho*Ss*Cl/2)*vx^2 + (1/4)*m*g; %-(1/4)*xdot_ref*thetadot_ref;
L4_ref = L1_ref;
L3_ref = (1/2)*((zA/xB)*(rho*Ss*Cd/2)*vx^2 - (xA/xB)*(rho*Ss*Cl/2)*vx^2 - (zB/xB)*(PR+PL) + 2*L1_ref);
L6_ref = L3_ref;
ir1_ref = sqrt( 1/(mu0*Nr^2*Al/4)*(L1_ref)*zi_ref^2 );
ir2_ref = sqrt( 1/(mu0*Nr^2*Al/4)*(L2_ref)*zi_ref^2 );
ir3_ref = sqrt( 1/(mu0*Nr^2*Al/4)*(L3_ref)*zi_ref^2 );
ir4_ref = sqrt( 1/(mu0*Nr^2*Al/4)*(L4_ref)*zi_ref^2 );
ir5_ref = sqrt( 1/(mu0*Nr^2*Al/4)*(L5_ref)*zi_ref^2 );
ir6_ref = sqrt( 1/(mu0*Nr^2*Al/4)*(L6_ref)*zi_ref^2 );


Vr1_ref = Rz*ir1_ref;
Vr2_ref = Rz*ir2_ref;
Vr3_ref = Rz*ir3_ref;
Vr4_ref = Rz*ir4_ref;
Vr5_ref = Rz*ir5_ref;
Vr6_ref = Rz*ir6_ref;

Zref(7)=ir1_ref;
Zref(8)=ir2_ref;
Zref(9)=ir3_ref;
Zref(10)=ir4_ref;
Zref(11)=ir5_ref;
Zref(12)=ir6_ref;

Vref_z = [Vr1_ref;Vr2_ref;Vr3_ref;Vr4_ref;Vr5_ref;Vr6_ref];
